simulink model "METI_Thermal_ver01_Jmaab_2018b"  (R2018b)
settings: Solver=ode8  StartTime=0  StopTime=end_time  FixedStep=sampling_time  RelTol=1e-3
PreLoadFcn:
  | %init_setting;
values from neighbouring files (symbols this model uses):
  degC2K = 273.15    [METI_TRAMI_Thermal_ver01_Jmaab_PreLoad.m]    (also in init_setting_METI.m)
  K2degC = -273.15    [METI_TRAMI_Thermal_ver01_Jmaab_PreLoad.m]    (also in init_setting_METI.m)
  sampling_time = 0.0025    [METI_TRAMI_Thermal_ver01_Jmaab_PreLoad.m]
undefined symbols (not defined in the file or in its folder): ACC_D_Gain, ACC_I_Gain, ACC_P_Gain, ALT_CNT_ALT_OFF_RPM_HYS_rpm, ALT_CNT_ALT_ON_RPM_HYS_rpm, ALT_CNT_Alter_V_BASE_V, ALT_CNT_Alter_V_Kaisei_V, ALT_CNT_flag_disable_kaisei, ALT_CNT_V_Battely_Kudo_V, ALT_PNT_ALT_GDCurrent_A, ALT_PNT_ALT_GDVolt_V, ALT_PNT_Alter_limit_Current_V_table, ALT_PNT_Alter_limit_Current_V_table_x_rpm, ALT_PNT_Alter_trq_Nm_map, ALT_PNT_Alter_trq_Nm_map_x_rpm, ALT_PNT_Alter_trq_Nm_map_y_Current_A, ALT_PNT_Alter_trq_Nm_map_z_Volt_tgt_V, ALT_PNT_eta_pulley_alt, ALT_PNT_Gain_Alt_v_del, ALT_PNT_ratio_pulley_alt, ALT_PNT_Tau_Alternator_V_tgt_s, ALT_PNT_trq_alter_output_LL_Nm, BK_PNT_Pow_UL, BK_PNT_Tau_brake, Brk_LL, Brk_PGain, Brk_UL, BT_PNT_Lo_Capa_lo_batt_F, BT_PNT_Lo_ocv_SOC_lo_batt_OCV_V_table, BT_PNT_Lo_ocv_SOC_lo_batt_OCV_V_table_x_SOC, BT_PNT_Lo_R_lo_batt_ohm, BT_PNT_Lo_SOC_MAX_lo_batt, BT_PNT_Lo_SOC_MIN_lo_batt, BT_PNT_Lo_SOC_START_lo_batt, BT_PNT_Lo_V_start_ocv, DF_PNT_DF_gear, DF_PNT_DFBlock2DFAir_Heat_Resi_KpW, DF_PNT_DFBlock_Heat_Capa_JpK, DF_PNT_DFBlock_Temp_ini_degC, DF_PNT_DFOil2DFBlock_Heat_Resi_KpW, DF_PNT_DFOil_Heat_Capa_JpK, DF_PNT_DFOil_Temp_ini_degC, DF_PNT_Driveshaft_damper, DF_PNT_Driveshaft_delta_radps_LL, DF_PNT_Driveshaft_delta_radps_UL, DF_PNT_Driveshaft_spring, DF_PNT_eta_DF, DF_PNT_Outtemp_degC, DF_PNT_TMBlock2DFBlock_Heat_Resi_KpW, Driver_Brake_Const1, Driver_Brake_Const3, Driver_Brake_Switch_Const2, Driver_Brk_sh, drivmode_ACC, drivmode_CONST, drivmode_GensokuKaisei, drivmode_GensokuRikko, drivmode_STOP, EL_PNT_R_bodyelec_lo_ohm, ENG_CNT_acc_idlestop ... (+137)
libraries: METI_Lib_vehicle_model x31, simulink x7, AZAPA_Lib_vehicle_model x1
(part 3 of 4)

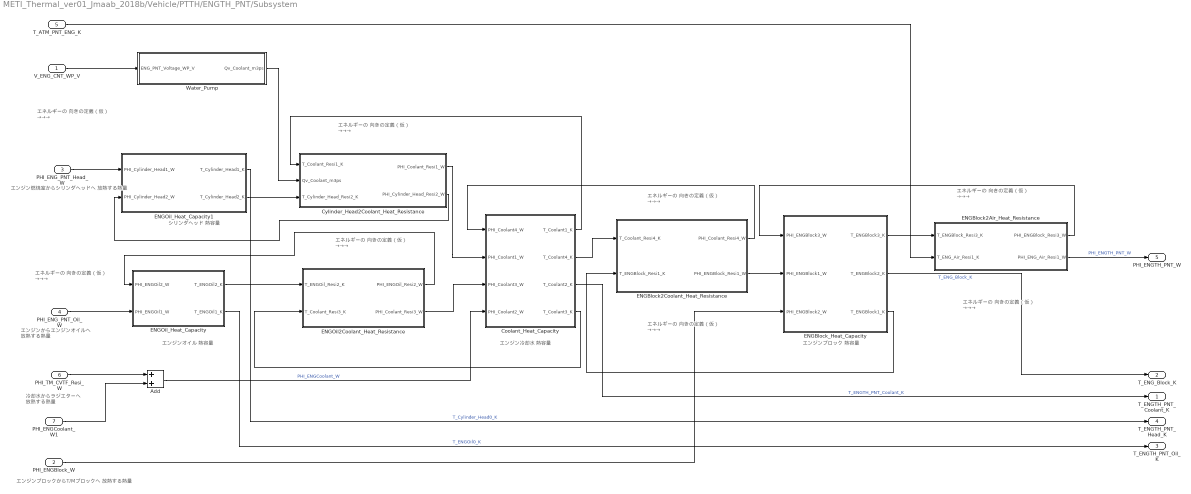
== system METI_Thermal_ver01_Jmaab_2018b/Vehicle/PTTH/ENGTH_PNT/Subsystem ==
  note: エンジンオイル
      | 熱容量
  note: エンジン冷却水
      | 熱容量
  note: エンジンブロック
      | 熱容量
  note: 冷却水からラジエターへ
      | 放熱する熱量
  note: エネルギーの
      | 向きの定義（仮）
      | →→→
  note: エンジン燃焼室からシリンダヘッドへ
      | 放熱する熱量
  note: エンジンからエンジンオイルへ
      | 放熱する熱量
  note: エネルギーの
      | 向きの定義（仮）
      | →→→
  note: エネルギーの
      | 向きの定義（仮）
      | →→→
  note: エネルギーの
      | 向きの定義（仮）
      | →→→
  note: エネルギーの
      | 向きの定義（仮）
      | →→→
  note: エネルギーの
      | 向きの定義（仮）
      | →→→
  note: エネルギーの
      | 向きの定義（仮）
      | →→→
  note: エンジンブロックからT/Mブロックへ
      | 放熱する熱量
  note: シリンダヘッド
      | 熱容量
  note: エネルギーの
      | 向きの定義（仮）
      | →→→
  V_ENG_CNT_WP_V : Inport
  PHI_ENGBlock_W : Inport  Port=2
  PHI_ENG_PNT_Head_W : Inport  Port=3
  PHI_ENG_PNT_Oil_W : Inport  Port=4
  T_ATM_PNT_ENG_K : Inport  Port=5
  PHI_TM_CVTF_Resi_W : Inport  Port=6
  PHI_ENGCoolant_W1 : Inport  Port=7
  Add : Sum
  Coolant_Heat_Capacity : Subsystem
  Cylinder_Head2Coolant_Heat_Resistance : Subsystem
  ENGBlock2Air_Heat_Resistance : Subsystem
  ENGBlock2Coolant_Heat_Resistance : Subsystem
  ENGBlock_Heat_Capacity : Subsystem
  ENGOil2Coolant_Heat_Resistance : Subsystem
  ENGOil_Heat_Capacity : Subsystem
  ENGOil_Heat_Capacity1 : Subsystem
  Water_Pump : Subsystem
  T_ENGTH_PNT_Coolant_K : Outport
  T_ENG_Block_K : Outport  Port=2
  T_ENGTH_PNT_Oil_K : Outport  Port=3
  T_ENGTH_PNT_Head_K : Outport  Port=4
  PHI_ENGTH_PNT_W : Outport  Port=5
  wires:
  PHI_TM_CVTF_Resi_W/1 -> Add/1
  Add/1 -> Coolant_Heat_Capacity/4(PHI_Coolant2_W)  "PHI_ENGCoolant_W"
  ENGOil_Heat_Capacity/1(T_ENGOil2_K) -> ENGOil2Coolant_Heat_Resistance/1(T_ENGOil_Resi2_K)
  ENGOil2Coolant_Heat_Resistance/2(PHI_Coolant_Resi3_W) -> Coolant_Heat_Capacity/3(PHI_Coolant3_W)
  PHI_ENGCoolant_W1/1 -> Add/2
  PHI_ENG_PNT_Head_W/1 -> ENGOil_Heat_Capacity1/1(PHI_Cylinder_Head1_W)
  ENGBlock_Heat_Capacity/3(T_ENGBlock1_K) -> ENGBlock2Coolant_Heat_Resistance/2(T_ENGBlock_Resi1_K)
  ENGBlock_Heat_Capacity/1(T_ENGBlock3_K) -> ENGBlock2Air_Heat_Resistance/1(T_ENGBlock_Resi3_K)
  ENGOil_Heat_Capacity1/1(T_Cylinder_Head1_K) -> T_ENGTH_PNT_Head_K/1  "T_Cylinder_Head0_K"
  Cylinder_Head2Coolant_Heat_Resistance/1(PHI_Coolant_Resi1_W) -> Coolant_Heat_Capacity/2(PHI_Coolant1_W)
  Cylinder_Head2Coolant_Heat_Resistance/2(PHI_Cylinder_Head_Resi2_W) -> ENGOil_Heat_Capacity1/2(PHI_Cylinder_Head2_W)
  Water_Pump/1(Qv_Coolant_m3ps) -> Cylinder_Head2Coolant_Heat_Resistance/2(Qv_Coolant_m3ps)
  ENGBlock_Heat_Capacity/2(T_ENGBlock2_K) -> T_ENG_Block_K/1  "T_ENG_Block_K"
  PHI_ENGBlock_W/1 -> ENGBlock_Heat_Capacity/3(PHI_ENGBlock2_W)
  V_ENG_CNT_WP_V/1 -> Water_Pump/1(ENG_PNT_Voltage_WP_V)
  ENGOil_Heat_Capacity1/2(T_Cylinder_Head2_K) -> Cylinder_Head2Coolant_Heat_Resistance/3(T_Cylinder_Head_Resi2_K)
  ENGBlock2Coolant_Heat_Resistance/1(PHI_Coolant_Resi4_W) -> Coolant_Heat_Capacity/1(PHI_Coolant4_W)
  Coolant_Heat_Capacity/4(T_Coolant3_K) -> ENGOil2Coolant_Heat_Resistance/2(T_Coolant_Resi3_K)
  ENGBlock2Air_Heat_Resistance/1(PHI_ENGBlock_Resi3_W) -> ENGBlock_Heat_Capacity/1(PHI_ENGBlock3_W)
  ENGOil2Coolant_Heat_Resistance/1(PHI_ENGOil_Resi2_W) -> ENGOil_Heat_Capacity/1(PHI_ENGOil2_W)
  Coolant_Heat_Capacity/2(T_Coolant4_K) -> ENGBlock2Coolant_Heat_Resistance/1(T_Coolant_Resi4_K)
  T_ATM_PNT_ENG_K/1 -> ENGBlock2Air_Heat_Resistance/2(T_ENG_Air_Resi1_K)
  ENGBlock2Coolant_Heat_Resistance/2(PHI_ENGBlock_Resi1_W) -> ENGBlock_Heat_Capacity/2(PHI_ENGBlock1_W)
  Coolant_Heat_Capacity/3(T_Coolant2_K) -> T_ENGTH_PNT_Coolant_K/1  "T_ENGTH_PNT_Coolant_K"
  Coolant_Heat_Capacity/1(T_Coolant1_K) -> Cylinder_Head2Coolant_Heat_Resistance/1(T_Coolant_Resi1_K)
  ENGBlock2Air_Heat_Resistance/2(PHI_ENG_Air_Resi1_W) -> PHI_ENGTH_PNT_W/1  "PHI_ENGTH_PNT_W"
  ENGOil_Heat_Capacity/2(T_ENGOil1_K) -> T_ENGTH_PNT_Oil_K/1  "T_ENGOil0_K"
  PHI_ENG_PNT_Oil_W/1 -> ENGOil_Heat_Capacity/2(PHI_ENGOil1_W)

== system METI_Thermal_ver01_Jmaab_2018b/Vehicle/PTTH/RDTH_PNT/Subsystem ==
  note: サーモスタット
  note: エネルギーの
      | 向きの定義（仮）
      | →→→
  note: エネルギーの
      | 向きの定義（仮）
      | →→→
  RD_PNT_Voltage_RDFan_V : Inport
  v_VL_PNT_kmph : Inport  Port=2
  T_ENGTH_PNT_Coolant_K : Inport  Port=3
  T_ATM_PNT_RD_K : Inport  Port=4
  ENGBlock2Coolant_Heat_Resistance : Subsystem
  RDCoolant2Air_Heat_Resistance : Subsystem
  RDCoolant_Heat_Capacity : Subsystem
  RD_Core_Heat_Resi_Calc : Subsystem
  T_RDCoolant_degC : Outport
  PHI_RDTH_PNT_W : Outport  Port=2
  PHI_RD_Air_Resi_W : Outport  Port=3
  tag scope: RD_PNT_RDCore_Heat_Resi_KpW=global
  wires:
  T_ATM_PNT_RD_K/1 -> RDCoolant2Air_Heat_Resistance/1(T_RD_Air_Resi_K)
  RDCoolant_Heat_Capacity/2(T_RDCoolant2_K) -> T_RDCoolant_degC/1, RDCoolant2Air_Heat_Resistance/3(T_RDCoolant_Resi2_K)  "T_RDCoolant_degC"
  RDCoolant_Heat_Capacity/1(T_RDCoolant1_K) -> ENGBlock2Coolant_Heat_Resistance/1(T_RDCoolant_Resi1_K)
  RD_Core_Heat_Resi_Calc/1("RD_PNT_RDCore_Heat_Resi_KpW ") -> [RD_PNT_RDCore_Heat_Resi_KpW], RDCoolant2Air_Heat_Resistance/2("RD_PNT_RDCore_Heat_Resi_KpW ")
  RDCoolant2Air_Heat_Resistance/1(PHI_RD_Air_Resi1_W) -> PHI_RD_Air_Resi_W/1  "PHI_RD_Air_Resi_W"
  T_ENGTH_PNT_Coolant_K/1 -> ENGBlock2Coolant_Heat_Resistance/2(T_Thermostat_Resi1_K)
  ENGBlock2Coolant_Heat_Resistance/2(PHI_Thermostat_Resi1_W) -> PHI_RDTH_PNT_W/1  "PHI_RDTH_PNT_W"
  RDCoolant2Air_Heat_Resistance/2(PHI_RDCoolant_Resi2_W) -> RDCoolant_Heat_Capacity/2(PHI_RDCoolant2_W)
  ENGBlock2Coolant_Heat_Resistance/1(PHI_RDCoolant_Resi1_W) -> RDCoolant_Heat_Capacity/1(PHI_RDCoolant1_W)
  RD_PNT_Voltage_RDFan_V/1 -> RD_Core_Heat_Resi_Calc/1(RD_PNT_Voltage_RDFan_V)
  v_VL_PNT_kmph/1 -> RD_Core_Heat_Resi_Calc/2(v_VL_PNT_kmph)

== system METI_Thermal_ver01_Jmaab_2018b/Vehicle/TM_PNT/DF_PNT/DriveShaft ==
  note: ドライブシャフトモデル
      | 硬いバネダンパー
  w_TR_PNT_radps : Inport
  w_DS_PNT_in_radps : Inport  Port=2
  Gain : Gain  Gain=-1
  Gain1 : Gain  Gain=DF_PNT_Driveshaft_spring
  Gain2 : Gain  Gain=DF_PNT_Driveshaft_damper
  Integrator : Integrator  LimitOutput=on  UpperSaturationLimit=DF_PNT_Driveshaft_delta_radps_UL  LowerSaturationLimit=DF_PNT_Driveshaft_delta_radps_LL
  Sum : Sum  Inputs=|+-
  Sum2 : Sum  Inputs=|++
  trq_DS_PNT_in_Nm : Outport
  trq_DF_PNT_Nm : Outport  Port=2
  wires:
  w_TR_PNT_radps/1 -> Sum/2
  w_DS_PNT_in_radps/1 -> Sum/1
  Integrator/1 -> Gain1/1
  Sum/1 -> Integrator/1, Gain2/1
  Gain1/1 -> Sum2/1
  Gain2/1 -> Sum2/2
  Sum2/1 -> Gain/1, trq_DS_PNT_in_Nm/1
  Gain/1 -> trq_DF_PNT_Nm/1

== system METI_Thermal_ver01_Jmaab_2018b/Vehicle/TM_PNT/TM_PNT/Flywheel ==
  trq_TM_PNT_in_Nm : Inport
  trq_TM_PNT_in_Nm1 : Inport  Port=2
  Divide : Product  Inputs=*/
  Inertia : Constant  Value=TM_PNT_Flywheel_Inertia_kgm2
  Integrator : Integrator  InitialCondition=TM_PNT_Flywheel_Init_radps  LimitOutput=on  LowerSaturationLimit=0
  P_cal : METI_Lib_vehicle_model/P_cal  Commented=on  Type_energy=回転運動  Type_output_energy=出力  Power_name=Po_  t_Workspace_Name=TM_PNT_Flywheel  P_VariableName=Po_TM_PNT_Flywheel  Across_VariableName=w_TM_PNT_Flywheel  Throgh_VariableName=tq_TM_PNT_Flywheel
  Sum : Sum  Inputs=|++
  Terminator : Terminator  Commented=on
  w_ENG_PNT_radps : Outport
  w_TM_PNT_in_radps : Outport  Port=2
  wires:
  Integrator/1 -> P_cal/1, w_TM_PNT_in_radps/1, w_ENG_PNT_radps/1
  trq_TM_PNT_in_Nm/1 -> Sum/1
  trq_TM_PNT_in_Nm1/1 -> Sum/2
  Inertia/1 -> Divide/2
  Sum/1 -> Divide/1, P_cal/2
  P_cal/1 -> Terminator/1
  Divide/1 -> Integrator/1

== system METI_Thermal_ver01_Jmaab_2018b/Vehicle/TM_PNT/TM_PNT/Inertia ==
  trq_TM_PNT_out_Nm0 : Inport
  trq_TM_PNT_Nm : Inport  Port=2
  Divide : Product  Inputs=*/
  Inertia : Constant  Value=TM_PNT_Driveshaft_Inertia_kgm2
  Integrator : Integrator  InitialCondition=000*(2*pi)/60  LimitOutput=on  LowerSaturationLimit=0
  P_cal : METI_Lib_vehicle_model/P_cal  Type_energy=回転運動  Type_output_energy=出力  Power_name=Po_  t_Workspace_Name=TM_PNT_inertia_MECK  P_VariableName=Po_TM_PNT_inertia_MECK  Across_VariableName=w_TM_PNT_inertia_MECK  Throgh_VariableName=tq_TM_PNT_inertia_MECK
  Sum : Sum  Inputs=|++
  Terminator : Terminator
  w_TM_PNT_out_radps : Outport
  w_TM_PNT_out_radps0 : Outport  Port=2
  wires:
  Integrator/1 -> P_cal/1, w_TM_PNT_out_radps0/1, w_TM_PNT_out_radps/1
  Divide/1 -> Integrator/1
  trq_TM_PNT_out_Nm0/1 -> Sum/1
  trq_TM_PNT_Nm/1 -> Sum/2
  Inertia/1 -> Divide/2
  Sum/1 -> Divide/1, P_cal/2
  P_cal/1 -> Terminator/1

== system METI_Thermal_ver01_Jmaab_2018b/Vehicle/TM_PNT/TM_PNT/K->degC6 ==
  K : Inport
  Constant2 : Constant  Value=K2degC
  Sum : Sum  Inputs=++|
  degC : Outport
  wires:
  K/1 -> Sum/2
  Constant2/1 -> Sum/1
  Sum/1 -> degC/1

== system METI_Thermal_ver01_Jmaab_2018b/Vehicle/TM_PNT/TM_PNT/TC_PNT ==
  note: ロックアップクラッチ
  note: トルクコンバータ
  flag_Lockup : Inport
  omg_Slip_rpm : Inport  Port=2
  w_TM_PNT_in_radps : Inport  Port=3
  w_TM_PNT_in_radps2 : Inport  Port=4
  Gain : Gain  Gain=-1
  LU_Clutch : Subsystem
  P_cal : METI_Lib_vehicle_model/P_cal  Type_energy=回転運動  Type_output_energy=出力  Power_name=Po_  t_Workspace_Name=TM_PNT_TC_MECK_UP  P_VariableName=Po_TM_PNT_TC_MECK_UP  Across_VariableName=w_TM_PNT_TC_MECK_UP  Throgh_VariableName=tq_TM_PNT_TC_MECK_UP
  P_cal1 : METI_Lib_vehicle_model/P_cal  Type_energy=回転運動  Type_output_energy=出力  Power_name=Po_  t_Workspace_Name=TM_PNT_TC_MECK_DN  P_VariableName=Po_TM_PNT_TC_MECK_DN  Across_VariableName=w_TM_PNT_TC_MECK_DN  Throgh_VariableName=tq_TM_PNT_TC_MECK_DN
  P_cal2 : METI_Lib_vehicle_model/P_cal  Type_energy=回転運動  Type_output_energy=出力  Power_name=Po_  t_Workspace_Name=TM_PNT_LU_MECK_UP  P_VariableName=Po_TM_PNT_LU_MECK_UP  Across_VariableName=w_TM_PNT_LU_MECK_UP  Throgh_VariableName=tq_TM_PNT_LU_MECK_UP
  P_cal3 : METI_Lib_vehicle_model/P_cal  Type_energy=回転運動  Type_output_energy=出力  Power_name=Po_  t_Workspace_Name=TM_PNT_LU_MECK_DN  P_VariableName=Po_TM_PNT_LU_MECK_DN  Across_VariableName=w_TM_PNT_LU_MECK_DN  Throgh_VariableName=tq_TM_PNT_LU_MECK_DN
  Sum : Sum  Inputs=|++
  Sum1 : Sum  Inputs=|++
  T_C : Subsystem
  Terminator{,1..4} (5 alike) : Terminator
  trq_TM_PNT_in_Nm2 : Outport
  trq_TM_PNT_in_Nm1 : Outport  Port=2
  wires:
  T_C/2(trq_TC_Nm2) -> Sum/2, P_cal/2
  w_TM_PNT_in_radps/1 -> T_C/1(w_TM_PNT_in_radps1), P_cal/1, LU_Clutch/2(w_TM_PNT_in_radps1), P_cal2/1
  Sum/1 -> Gain/1
  T_C/1(trq_TC_Nm1) -> P_cal1/2, Sum1/2
  Sum1/1 -> trq_TM_PNT_in_Nm2/1
  w_TM_PNT_in_radps2/1 -> LU_Clutch/3(w_TM_PNT_in_radps2), P_cal1/1, P_cal3/1, T_C/2(w_TM_PNT_in_radps2)
  P_cal/1 -> Terminator/1
  P_cal1/1 -> Terminator1/1
  omg_Slip_rpm/1 -> Terminator3/1
  LU_Clutch/1(trq_LUC_Nm1) -> Sum/1, P_cal2/2
  LU_Clutch/2(trq_LUC_Nm2) -> Sum1/1, P_cal3/2
  flag_Lockup/1 -> LU_Clutch/1(LockUP_Signal)
  P_cal2/1 -> Terminator2/1
  P_cal3/1 -> Terminator4/1
  Gain/1 -> trq_TM_PNT_in_Nm1/1

== system METI_Thermal_ver01_Jmaab_2018b/Vehicle/TM_PNT/TM_PNT/VR_PNT ==
  note: ギア比変換
  ratio_CVT : Inport
  trq_TM_PNT_in_Nm2 : Inport  Port=2
  w_TM_PNT_out_radps0 : Inport  Port=3
  T_TMTH_PNT_CVTF_dC : Inport  Port=4
  1-D Lookup Table : Lookup_n-D  NumberOfTableDimensions=1  BreakpointsForDimension1=TM_PNT_eta_CVT_x_CVTF_degC  Table=TM_PNT_eta_CVT  InternalRulePriority=Speed  RndMeth=Simplest  InputSameDT=on
  Goto1 : Goto  Commented=on  GotoTag=trq_Variator_Nm
  P_cal : METI_Lib_vehicle_model/P_cal  Type_energy=回転運動  Type_output_energy=損失  Power_name=Pl_  t_Workspace_Name=TM_PNT_Variator_MECK_LOSS  P_VariableName=Pl_TM_PNT_Variator_MECK_LOSS  Across_VariableName=w_TM_PNT_Variator_MECK_LOSS  Throgh_VariableName=tq_TM_PNT_Variator_MECK_LOSS
  Product : Product  RndMeth=Zero
  Product1 : Product  RndMeth=Zero
  Transfer Fcn : TransferFcn  Denominator=[TM_PNT_Tau_CVT_ratio_s 1]
  eta_cal_CVT : METI_Lib_vehicle_model/eta_cal_InHi  SystemSampleTime=-1
  trq_TM_PNT_out_Nm0 : Outport
  w_TM_PNT_in_radps2 : Outport  Port=2
  tag scope: tScope_CVTLoss=global
  wires:
  trq_TM_PNT_in_Nm2/1 -> eta_cal_CVT/2
  Product/1 -> w_TM_PNT_in_radps2/1, P_cal/1
  w_TM_PNT_out_radps0/1 -> Product/2
  ratio_CVT/1 -> Transfer Fcn/1
  Product1/1 -> Goto1/1, trq_TM_PNT_out_Nm0/1
  eta_cal_CVT/2 -> Product1/2
  P_cal/1 -> [tScope_CVTLoss]
  Transfer Fcn/1 -> Product1/1, Product/1
  1-D Lookup Table/1 -> eta_cal_CVT/1
  eta_cal_CVT/1 -> P_cal/2
  T_TMTH_PNT_CVTF_dC/1 -> 1-D Lookup Table/1

== system METI_Thermal_ver01_Jmaab_2018b/Driver/Caliculate_Opeining_Accel/FF/Cal_M_ENG_jiku2/Subsystem ==
  In1 : Inport
  Constant1 : Constant  Value=0
  Switch : Switch  Criteria=u2 > Threshold  Threshold=0.1
  Out1 : Outport
  wires:
  Switch/1 -> Out1/1
  Constant1/1 -> Switch/3
  In1/1 -> Switch/2, Switch/1

== system METI_Thermal_ver01_Jmaab_2018b/Vehicle/ALT_PNT/Subsystem/I_alt_cal/Cal_I_alt_P_control ==
  note: 目標電圧よりもオルタネータ電圧が低い場合電流をPI制御で出力
      | 高い場合は、電流を0とする
  V_delt_tgt : Inport
  Gain : Gain  Gain=ALT_PNT_Gain_Alt_v_del
  Transfer Fcn : TransferFcn  Denominator=[ALT_PNT_Tau_Alternator_V_tgt_s 1]
  I_alt_base : Outport
  wires:
  Gain/1 -> I_alt_base/1
  V_delt_tgt/1 -> Transfer Fcn/1
  Transfer Fcn/1 -> Gain/1

== system METI_Thermal_ver01_Jmaab_2018b/Vehicle/ALT_PNT/Subsystem/I_alt_cal/Cal_I_alt_base ==
  note: 目標電圧よりもオルタネータ電圧が低い場合電流をPI制御で出力
      | 高い場合は、電流を0とする
  V_delt_tgt : Inport
  Constant : Constant  Value=0
  Gain : Gain  Gain=1/BT_PNT_Lo_R_lo_batt_ohm
  MinMax : MinMax  Function=max  Inputs=2
  Switch : Switch  Criteria=u2 > Threshold
  Transfer Fcn : TransferFcn  Denominator=[ALT_PNT_Tau_Alternator_V_tgt_s 1]
  I_alt_base : Outport
  wires:
  MinMax/1 -> I_alt_base/1
  Gain/1 -> Switch/1
  V_delt_tgt/1 -> Transfer Fcn/1
  Constant/1 -> MinMax/2, Switch/3
  Switch/1 -> MinMax/1
  Transfer Fcn/1 -> Switch/2, Gain/1

== system METI_Thermal_ver01_Jmaab_2018b/Vehicle/CNT/ENG_CNT/ENG_Cntrl/Caliculate_Idle_Speed ==
  note: 目標アイドル回転数
  note: ○目標回転数に対するP制御
  note: 補機負荷やNDの時の負荷によるアイドル安定化処理を入れる
      | パワーデマンドで締結
  per_throttle_base : Inport
  n_eng_rpm : Inport  Port=2
  flag_Lockup : Inport  Port=3
  flag_IdleStop : Inport  Port=4
  T_ENGTH_PNT_Coolant_dC : Inport  Port=5
  Subsystem : Subsystem
  Subsystem1 : Subsystem
  Subtract : Sum  Inputs=+-
  Tw2ENG_CNT_IdleSpeed : Lookup_n-D  NumberOfTableDimensions=1  BreakpointsForDimension1=T_ENGCoodant_T_ENGCoodant  Table=ENG_CNT_IdleSpeed  InternalRulePriority=Speed  RndMeth=Simplest  InputSameDT=on
  per_isc_[%] : Outport
  tag scope: ENG_CNT_IdleSpeed=global
  wires:
  n_eng_rpm/1 -> Subsystem1/2(n_eng_rpm), Subtract/2
  Subtract/1 -> Subsystem/1(del_omg_engine)
  per_throttle_base/1 -> Subsystem1/3(per_throttle_base)
  flag_Lockup/1 -> Subsystem1/4(flag_Lockup)
  Subsystem1/1(flag_idle_fb) -> Subsystem/2(flag_idle_fb)
  flag_IdleStop/1 -> Subsystem1/5(flag_IdleStop)
  Subsystem/1(per_isc_[%]) -> per_isc_[%]/1
  T_ENGTH_PNT_Coolant_dC/1 -> Tw2ENG_CNT_IdleSpeed/1
  Tw2ENG_CNT_IdleSpeed/1 -> [ENG_CNT_IdleSpeed], Subsystem1/1(omg_tgt_idle), Subtract/1

== system METI_Thermal_ver01_Jmaab_2018b/Vehicle/CNT/ENG_CNT/ENG_Cntrl/Injection_Control ==
  T_ENGTH_PNT_Coolant_dC : Inport
  Tw2KFuel : Lookup_n-D  NumberOfTableDimensions=1  BreakpointsForDimension1=T_ENGCoodant  Table=K_Fuel  RndMeth=Simplest  InputSameDT=on
  K_Fuel : Outport
  wires:
  Tw2KFuel/1 -> K_Fuel/1  "K_Fuel"
  T_ENGTH_PNT_Coolant_dC/1 -> Tw2KFuel/1

== system METI_Thermal_ver01_Jmaab_2018b/Vehicle/CNT/ENG_CNT/ENG_Cntrl/K->degC7 ==
  K : Inport
  Constant2 : Constant  Value=K2degC
  Sum : Sum  Inputs=++|
  degC : Outport
  wires:
  Sum/1 -> degC/1
  Constant2/1 -> Sum/1
  K/1 -> Sum/2

== system METI_Thermal_ver01_Jmaab_2018b/Vehicle/CNT/ENG_CNT/ENG_Cntrl/RD_Fan_Control ==
  T_ENGTH_PNT_Coolant_dC : Inport
  1-D Lookup Table1 : Lookup_n-D  NumberOfTableDimensions=1  BreakpointsForDimension1=ENG_CNT_V_RDFan_x_T_Coolant  BeginIndexSearchUsingPreviousIndexResult=on  Table=ENG_CNT_V_RDFan_V  InternalRulePriority=Speed  RndMeth=Simplest  InputSameDT=on
  V_RDTH_PNT_Fan_V : Outport
  wires:
  T_ENGTH_PNT_Coolant_dC/1 -> 1-D Lookup Table1/1
  1-D Lookup Table1/1 -> V_RDTH_PNT_Fan_V/1

== system METI_Thermal_ver01_Jmaab_2018b/Vehicle/CNT/ENG_CNT/ENG_Cntrl/Set_Fuel_Cut ==
  note: ○減速時のフューエルカット条件
      | 　・停車中でない
      | 　・回転数がある回転数以上
      | 　・アクセル開度がOFF
  v_vehicle : Inport
  n_eng_rpm : Inport  Port=2
  per_throttle_base : Inport  Port=3
  Constant1 : Constant  Value=ENG_CNT_V_vhicle_fuelcut_kmph
  Constant4 : Constant  Value=ENG_CNT_omg_eng_fuelcut_rpm
  Constant6 : Constant  Value=ENG_CNT_per_throttle_fuelcut
  Logical Operator : Logic  Inputs=3  AllPortsSameDT=off  OutDataTypeStr=boolean
  Relational Operator1 : RelationalOperator  Operator=<=  OutDataTypeStr=boolean  RndMeth=Nearest
  Relational Operator2 : RelationalOperator  OutDataTypeStr=boolean  RndMeth=Nearest
  Relational Operator3 : RelationalOperator  OutDataTypeStr=boolean  RndMeth=Nearest
  flag_fuelcut : Outport
  wires:
  n_eng_rpm/1 -> Relational Operator2/1
  per_throttle_base/1 -> Relational Operator1/1
  Constant6/1 -> Relational Operator1/2
  Relational Operator1/1 -> Logical Operator/3
  Relational Operator2/1 -> Logical Operator/2
  Logical Operator/1 -> flag_fuelcut/1
  Constant1/1 -> Relational Operator3/2
  v_vehicle/1 -> Relational Operator3/1
  Relational Operator3/1 -> Logical Operator/1
  Constant4/1 -> Relational Operator2/2

== system METI_Thermal_ver01_Jmaab_2018b/Vehicle/CNT/ENG_CNT/ENG_Cntrl/Set_Idle_Stop ==
  note: ○アイドリングストップ制御
      | 　停車時＋ブレーキを踏んでいるとき、アイドリングストップ
  open_accel_per : Inport
  v_vehicle : Inport  Port=2
  per_brake : Inport  Port=3
  T_ENGTH_PNT_Coolant_dC : Inport  Port=4
  Constant : Constant  Value=ENG_CNT_V_car_idlestop_kmph
  Constant1 : Constant  Value=ENG_CNT_brak_idlestop
  Constant2 : Constant  Value=ENG_CNT_flag_idle_stop_exe
  Constant3 : Constant  Value=ENG_CNT_acc_idlestop
  Logical Operator : Logic  Inputs=5  AllPortsSameDT=off  OutDataTypeStr=boolean
  Relational Operator : RelationalOperator  Operator=<  OutDataTypeStr=boolean  RndMeth=Nearest
  Relational Operator1 : RelationalOperator  OutDataTypeStr=boolean  RndMeth=Nearest
  Relational Operator2 : RelationalOperator  Operator=<  OutDataTypeStr=boolean  RndMeth=Nearest
  Relay : Relay  OnSwitchValue=ENG_CNT_IdleStop_flag_const  OffSwitchValue=ENG_CNT_IdleStop_flag_const-5
  flag_IdleStop : Outport
  wires:
  Relational Operator/1 -> Logical Operator/2
  Logical Operator/1 -> flag_IdleStop/1
  v_vehicle/1 -> Relational Operator/1
  per_brake/1 -> Relational Operator1/1
  Constant/1 -> Relational Operator/2
  Constant1/1 -> Relational Operator1/2
  Relational Operator1/1 -> Logical Operator/3
  Constant2/1 -> Logical Operator/1
  T_ENGTH_PNT_Coolant_dC/1 -> Relay/1
  Relay/1 -> Logical Operator/4
  open_accel_per/1 -> Relational Operator2/1
  Constant3/1 -> Relational Operator2/2
  Relational Operator2/1 -> Logical Operator/5

== system METI_Thermal_ver01_Jmaab_2018b/Vehicle/CNT/ENG_CNT/ENG_Cntrl/Starter ==
  note: サンプリング時間
  note: 時間リセット
  note: アイドリングフラグがON→OFFに
      | 切り替わり時スターターON開始
  note: スタータ開始時間
  note: スタータ開始時間から
      | ある時間超えたらOFF
  note: アイドリングフラグがON→OFFに切り替わり時スターターON開始.ある時間を超えたらOFF
  flag_idlestop : Inport
  n_eng_rpm : Inport  Port=2
  Constant2 : Constant  Value=ENG_CNT_Starter_timer_Const_s
  Constant4 : Constant  Value=sampling_time
  Constant5 : Constant  Value=0
  Constant6 : Constant  Value=OFF
  Constant7 : Constant  Value=ON
  IdleSpeed : Constant  Value=ENG_CNT_IdleSpeed_Const/2
  Logical Operator : Logic  Inputs=3  AllPortsSameDT=off  OutDataTypeStr=boolean
  Logical Operator1 : Logic  Operator=NOT  AllPortsSameDT=off  OutDataTypeStr=boolean
  Memory : Memory  InitialCondition=1000
  Memory1 : Memory  InheritSampleTime=on
  Relational Operator1 : RelationalOperator  Operator=<=  OutDataTypeStr=boolean  RndMeth=Nearest
  Relational Operator2 : RelationalOperator  Operator=<  OutDataTypeStr=boolean  RndMeth=Nearest
  Sum5 : Sum  Inputs=|++
  Switch3 : Switch  Criteria=u2 > Threshold  Threshold=0.5
  Switch4 : Switch  Criteria=u2 > Threshold  Threshold=0.5
  flag_ON_Starter : Outport
  wires:
  Switch4/1 -> flag_ON_Starter/1
  Memory/1 -> Sum5/2
  Constant4/1 -> Sum5/1
  Constant5/1 -> Switch3/1
  Sum5/1 -> Switch3/3
  Switch3/1 -> Relational Operator1/1, Memory/1
  Memory1/1 -> Logical Operator/2
  Logical Operator1/1 -> Logical Operator/1
  flag_idlestop/1 -> Memory1/1, Logical Operator1/1
  Logical Operator/1 -> Switch3/2
  Constant2/1 -> Relational Operator1/2
  Relational Operator1/1 -> Switch4/2
  Constant7/1 -> Switch4/1
  Constant6/1 -> Switch4/3
  n_eng_rpm/1 -> Relational Operator2/1
  IdleSpeed/1 -> Relational Operator2/2
  Relational Operator2/1 -> Logical Operator/3

== system METI_Thermal_ver01_Jmaab_2018b/Vehicle/CNT/ENG_CNT/ENG_Cntrl/Water_Pump_Control ==
  T_ENGTH_PNT_Coolant_dC : Inport
  1-D Lookup Table1 : Lookup_n-D  NumberOfTableDimensions=1  BreakpointsForDimension1=ENG_CNT_V_Water_Pump_x_T_Coolant  BeginIndexSearchUsingPreviousIndexResult=on  Table=ENG_CNT_V_Water_Pump_V  InternalRulePriority=Speed  RndMeth=Simplest  InputSameDT=on
  V_ENG_PNT_WP_V : Outport
  wires:
  T_ENGTH_PNT_Coolant_dC/1 -> 1-D Lookup Table1/1
  1-D Lookup Table1/1 -> V_ENG_PNT_WP_V/1

== system METI_Thermal_ver01_Jmaab_2018b/Vehicle/CNT/TM_CNT/TM_Ctrl/CVT_ECU ==
  per_throttle : Inport
  omg_pera : Inport  Port=2
  1-D Lookup Table : Lookup_n-D  NumberOfTableDimensions=1  BreakpointsForDimension1=TM_CNT_CVTpritgt_rpm_table_x_TVO  Table=TM_CNT_CVTpritgt_rpm_table  RndMeth=Simplest  InputSameDT=on
  Constant2 : Constant  Value=TM_CNT_CVT_radpmin_min_rpm
  Divide : Product  Inputs=*/
  Gain2 : Gain  Gain=TM_CNT_Gain_CVT_ECU
  HighestRatio : Constant  Value=TM_CNT_CVT_ratio_LL
  LowestRatio : Constant  Value=TM_CNT_CVT_ratio_UL
  MinMax : MinMax  Function=max  Inputs=2
  Saturation : Saturate  UpperLimit=TM_CNT_delta_CVT_ratio_UL  LowerLimit=TM_CNT_delta_CVT_ratio_LL
  Saturation Dynamic : simulink/Discontinuities/Saturation Dynamic  OutMin=[]  OutMax=[]  OutDataTypeStr=Inherit: Same as second input  OutDataType=fixdt(1, 16)  OutScaling=2^-10  DoSatur=off
  Sum : Sum  Inputs=|+-
  Sum1 : Sum  Inputs=|++
  Unit Delay : UnitDelay  InitialCondition=1  SampleTime=-1
  ratio_CVT : Outport
  wires:
  1-D Lookup Table/1 -> Divide/1
  Divide/1 -> Saturation Dynamic/2
  LowestRatio/1 -> Saturation Dynamic/1
  HighestRatio/1 -> Saturation Dynamic/3
  MinMax/1 -> Divide/2
  Saturation Dynamic/1 -> Sum/1
  Unit Delay/1 -> Sum1/2, Sum/2
  Sum1/1 -> ratio_CVT/1, Unit Delay/1
  Sum/1 -> Gain2/1
  Gain2/1 -> Saturation/1
  per_throttle/1 -> 1-D Lookup Table/1
  omg_pera/1 -> MinMax/2
  Saturation/1 -> Sum1/1
  Constant2/1 -> MinMax/1

== system METI_Thermal_ver01_Jmaab_2018b/Vehicle/CNT/TM_CNT/TM_Ctrl/K->degC ==
  K : Inport
  Constant2 : Constant  Value=K2degC
  Sum : Sum  Inputs=++|
  degC : Outport
  wires:
  Sum/1 -> degC/1
  Constant2/1 -> Sum/1
  K/1 -> Sum/2

== system METI_Thermal_ver01_Jmaab_2018b/Vehicle/CNT/TM_CNT/TM_Ctrl/K->degC1 ==
  K : Inport
  Constant2 : Constant  Value=K2degC
  Sum : Sum  Inputs=++|
  degC : Outport
  wires:
  K/1 -> Sum/2
  Constant2/1 -> Sum/1
  Sum/1 -> degC/1

== system METI_Thermal_ver01_Jmaab_2018b/Vehicle/CNT/TM_CNT/TM_Ctrl/LockupClutch_ECU ==
  v_vehicle : Inport
  per_throttle : Inport  Port=2
  2-D Lookup Table : Lookup_n-D  BreakpointsForDimension1=TM_CNT_LU_slip_rpm_map_y_TVO  BreakpointsForDimension2=TM_CNT_LU_slip_rpm_map_x_speed_kmph  Table=TM_CNT_LU_slip_rpm_map  RndMeth=Simplest  InputSameDT=on
  Relay : Relay  OnSwitchValue=TM_CNT_LU_Clutch_RelayON_rpm  OffSwitchValue=TM_CNT_LU_Clutch_RelayOFF_rpm  OnOutputValue=0  OffOutputValue=1
  flag_Lockup : Outport
  omg_Slip_rpm : Outport  Port=2
  wires:
  v_vehicle/1 -> 2-D Lookup Table/2
  2-D Lookup Table/1 -> omg_Slip_rpm/1, Relay/1
  per_throttle/1 -> 2-D Lookup Table/1
  Relay/1 -> flag_Lockup/1

== system METI_Thermal_ver01_Jmaab_2018b/Vehicle/CNT/TM_CNT/TM_Ctrl/WarmerECU ==
  note: ENG冷却水温＞CVTF温度
      | の時にこのマップを使用する
  note: CVTF温度が熱い時に
      | このマップを使用する
  T_TMTH_PNT_CVTF_dC : Inport
  T_ENG_Coolant_dC : Inport  Port=2
  1-D Lookup Table1 : Lookup_n-D  NumberOfTableDimensions=1  BreakpointsForDimension1=TM_CNT_CVTFwarmer_KpW_x_T_ENGCoolant  BeginIndexSearchUsingPreviousIndexResult=on  Table=TM_CNT_CVTFwarmer_KpW  ExtrapMethod=Clip  InternalRulePriority=Speed  RndMeth=Simplest  InputSameDT=on
  1-D Lookup Table2 : Lookup_n-D  NumberOfTableDimensions=1  BreakpointsForDimension1=TM_CNT_CVTFwarmer2_KpW_x_T_CVTF  BeginIndexSearchUsingPreviousIndexResult=on  Table=TM_CNT_CVTFwarmer2_KpW  ExtrapMethod=Clip  InternalRulePriority=Speed  RndMeth=Simplest  InputSameDT=on
  Add1 : Sum  Inputs=+-
  Compare To Zero1 : simulink/Logic and Bit Operations/Compare To Zero  relop=>  OutDataTypeStr=boolean
  Constant1 : Constant  Value=TM_CNT_CVTFwarmer_cold_Coolant_KpW
  MinMax : MinMax  Inputs=2
  Switch1 : Switch  Criteria=u2 > Threshold
  R_CVTF_warmer_tgt_KpW : Outport
  wires:
  MinMax/1 -> R_CVTF_warmer_tgt_KpW/1
  Add1/1 -> Compare To Zero1/1
  Compare To Zero1/1 -> Switch1/2
  1-D Lookup Table1/1 -> Switch1/1
  Constant1/1 -> Switch1/3
  T_ENG_Coolant_dC/1 -> 1-D Lookup Table1/1, Add1/1
  T_TMTH_PNT_CVTF_dC/1 -> 1-D Lookup Table2/1, Add1/2
  Switch1/1 -> MinMax/1
  1-D Lookup Table2/1 -> MinMax/2

== system METI_Thermal_ver01_Jmaab_2018b/Vehicle/ENG_PNT/ENG_Plant/Cal_FuelComsunption/Not_cal1 ==
  In1 : Inport
  Constant : Constant  Value=0
  Constant1 : Constant
  Switch : Switch  Criteria=u2 > Threshold  Threshold=0.5
  Out1 : Outport
  wires:
  Constant1/1 -> Switch/3
  Constant/1 -> Switch/1
  Switch/1 -> Out1/1
  In1/1 -> Switch/2

== system METI_Thermal_ver01_Jmaab_2018b/Vehicle/ENG_PNT/ENG_Plant/Cal_FuelComsunption/Not_cal2 ==
  In1 : Inport
  Constant : Constant  Value=0
  Constant1 : Constant
  Switch : Switch  Criteria=u2 > Threshold  Threshold=0.5
  Out1 : Outport
  wires:
  In1/1 -> Switch/2
  Switch/1 -> Out1/1
  Constant/1 -> Switch/1
  Constant1/1 -> Switch/3

== system METI_Thermal_ver01_Jmaab_2018b/Vehicle/ENG_PNT/ENG_Plant/Cal_trq_ENG_jiku/Not_cal ==
  In1 : Inport
  Constant : Constant  Value=0
  Constant1 : Constant
  Switch : Switch  Criteria=u2 > Threshold  Threshold=0.5
  Out1 : Outport
  wires:
  In1/1 -> Switch/2
  Switch/1 -> Out1/1
  Constant/1 -> Switch/1
  Constant1/1 -> Switch/3

== system METI_Thermal_ver01_Jmaab_2018b/Vehicle/ENG_PNT/ENG_Plant/Cal_trq_ENG_jiku/Not_cal1 ==
  In1 : Inport
  Constant : Constant  Value=0
  Constant1 : Constant
  Switch : Switch  Criteria=u2 > Threshold  Threshold=0.5
  Out1 : Outport
  wires:
  Constant1/1 -> Switch/3
  Constant/1 -> Switch/1
  Switch/1 -> Out1/1
  In1/1 -> Switch/2

== system METI_Thermal_ver01_Jmaab_2018b/Vehicle/PTTH/DTTH_PNT/DFTH_PNT/DFBlock_Heat_Capacity ==
  PHI_DFBlock3_W : Inport
  PHI_DFBlock2_W : Inport  Port=2
  PHI_DFBlock1_W : Inport  Port=3
  Add : Sum  Inputs=+++
  Add1 : Sum
  Constant : Constant  Value=DF_PNT_DFBlock_Heat_Capa_JpK
  Constant1 : Constant  Value=DF_PNT_DFBlock_Temp_ini_degC
  Divide : Product  Inputs=/*
  Integrator : Integrator
  degC->K : Subsystem
  T_DFBlock2_K : Outport
  T_DFBlock3_K : Outport  Port=2
  T_DFBlock1_K : Outport  Port=3
  wires:
  PHI_DFBlock1_W/1 -> Add/1
  Constant/1 -> Divide/1
  Add/1 -> Divide/2
  Divide/1 -> Integrator/1
  Integrator/1 -> Add1/2
  Add1/1 -> T_DFBlock1_K/1, T_DFBlock3_K/1, T_DFBlock2_K/1
  PHI_DFBlock2_W/1 -> Add/2
  PHI_DFBlock3_W/1 -> Add/3
  Constant1/1 -> degC->K/1(degC)
  degC->K/1(K) -> Add1/1

== system METI_Thermal_ver01_Jmaab_2018b/Vehicle/PTTH/DTTH_PNT/DFTH_PNT/DFOil2DFBlock_Heat_Resistance ==
  T_DFOil_Resi2_K : Inport
  T_DFBlock_Resi_K : Inport  Port=2
  Add : Sum  Inputs=+-
  Constant : Constant  Value=DF_PNT_DFOil2DFBlock_Heat_Resi_KpW
  Divide : Product  Inputs=*/
  Gain : Gain  Gain=-1
  Gain1 : Gain
  PHI_DFOil_Resi2_W : Outport
  PHI_DFBlock_Resi_W : Outport  Port=2
  wires:
  Constant/1 -> Divide/2
  Add/1 -> Divide/1
  Divide/1 -> Gain/1, Gain1/1
  Gain/1 -> PHI_DFOil_Resi2_W/1
  T_DFOil_Resi2_K/1 -> Add/1
  T_DFBlock_Resi_K/1 -> Add/2
  Gain1/1 -> PHI_DFBlock_Resi_W/1

== system METI_Thermal_ver01_Jmaab_2018b/Vehicle/PTTH/DTTH_PNT/DFTH_PNT/DFOil_Heat_Capacity ==
  PHI_DFOil2_W : Inport
  PHI_DFOil1_W : Inport  Port=2
  Add : Sum
  Add1 : Sum
  Constant : Constant  Value=DF_PNT_DFOil_Heat_Capa_JpK
  Constant1 : Constant  Value=DF_PNT_DFOil_Temp_ini_degC
  Divide : Product  Inputs=/*
  Integrator : Integrator
  degC->K : Subsystem
  T_DFOil2_K : Outport
  T_DFOil1_K : Outport  Port=2
  wires:
  PHI_DFOil2_W/1 -> Add/2
  PHI_DFOil1_W/1 -> Add/1
  Constant/1 -> Divide/1
  Add/1 -> Divide/2
  Divide/1 -> Integrator/1
  Integrator/1 -> Add1/2
  Add1/1 -> T_DFOil1_K/1, T_DFOil2_K/1
  Constant1/1 -> degC->K/1(degC)
  degC->K/1(K) -> Add1/1

== system METI_Thermal_ver01_Jmaab_2018b/Vehicle/PTTH/DTTH_PNT/DFTH_PNT/ENGBlock2Air_Heat_Resistance ==
  T_DFBlock_Resi_K : Inport
  T_DF_Air_Resi_K : Inport  Port=2
  Add : Sum  Inputs=+-
  Constant : Constant  Value=DF_PNT_DFBlock2DFAir_Heat_Resi_KpW
  Divide : Product  Inputs=*/
  Gain : Gain  Gain=-1
  Gain1 : Gain
  PHI_DFBlock_Resi_W : Outport
  PHI_DF_Air_Resi_W : Outport  Port=2
  wires:
  Constant/1 -> Divide/2
  Add/1 -> Divide/1
  Divide/1 -> Gain/1, Gain1/1
  Gain/1 -> PHI_DFBlock_Resi_W/1
  T_DFBlock_Resi_K/1 -> Add/1
  T_DF_Air_Resi_K/1 -> Add/2
  Gain1/1 -> PHI_DF_Air_Resi_W/1

== system METI_Thermal_ver01_Jmaab_2018b/Vehicle/PTTH/DTTH_PNT/DFTH_PNT/TMBlock2DFBlock_Heat_Resistance ==
  T_DFBlock_Resi_K : Inport
  T_TMBlock_Resi_K : Inport  Port=2
  Add : Sum  Inputs=+-
  Constant : Constant  Value=DF_PNT_TMBlock2DFBlock_Heat_Resi_KpW
  Divide : Product  Inputs=*/
  Gain : Gain  Gain=-1
  Gain1 : Gain
  PHI_DFBlock_Resi_W : Outport
  PHI_TMBlock_Resi_W : Outport  Port=2
  wires:
  Constant/1 -> Divide/2
  Add/1 -> Divide/1
  Divide/1 -> Gain/1, Gain1/1
  Gain/1 -> PHI_TMBlock_Resi_W/1
  T_TMBlock_Resi_K/1 -> Add/1
  T_DFBlock_Resi_K/1 -> Add/2
  Gain1/1 -> PHI_DFBlock_Resi_W/1

== system METI_Thermal_ver01_Jmaab_2018b/Vehicle/PTTH/DTTH_PNT/TMTH_PNT/CVTF2Coolant_Heat_Resistance ==
  note: エネルギーの
      | 向きの定義（仮）
      | ← ←←
  T_CVTF_Resi2_K : Inport
  R_CVTF_warmer_tgt_KpW : Inport  Port=2
  T_Coolant_Resi2_K : Inport  Port=3
  Add : Sum  Inputs=+-
  Divide : Product  Inputs=*/
  Gain : Gain  Gain=-1
  Gain1 : Gain  Gain=-1
  PHI_Coolant_Resi2_W : Outport
  PHI_CVTF_Resi2_W : Outport  Port=2
  wires:
  R_CVTF_warmer_tgt_KpW/1 -> Divide/2
  Add/1 -> Divide/1
  Divide/1 -> Gain/1, Gain1/1
  T_Coolant_Resi2_K/1 -> Add/2
  T_CVTF_Resi2_K/1 -> Add/1
  Gain/1 -> PHI_CVTF_Resi2_W/1
  Gain1/1 -> PHI_Coolant_Resi2_W/1

== system METI_Thermal_ver01_Jmaab_2018b/Vehicle/PTTH/DTTH_PNT/TMTH_PNT/CVTF2TMBlock_Heat_Resistance ==
  T_CVTF_Resi4_K : Inport
  T_TMBlock_Resi1_K : Inport  Port=2
  Add : Sum  Inputs=+-
  Constant : Constant  Value=TM_PNT_CVTF2TMBlock_Heat_Resi_KpW
  Divide : Product  Inputs=*/
  Gain : Gain  Gain=-1
  Gain1 : Gain
  PHI_CVTF_Resi4_W : Outport
  PHI_TMBlock_Resi1_W : Outport  Port=2
  wires:
  Constant/1 -> Divide/2
  Add/1 -> Divide/1
  Divide/1 -> Gain/1, Gain1/1
  Gain/1 -> PHI_CVTF_Resi4_W/1
  T_CVTF_Resi4_K/1 -> Add/1
  T_TMBlock_Resi1_K/1 -> Add/2
  Gain1/1 -> PHI_TMBlock_Resi1_W/1

== system METI_Thermal_ver01_Jmaab_2018b/Vehicle/PTTH/DTTH_PNT/TMTH_PNT/CVTF_Heat_Capacity ==
  PHI_CVTF4_W : Inport
  PHI_CVTF1_W : Inport  Port=2
  PHI_CVT2_W : Inport  Port=3
  Add : Sum  Inputs=+++
  Add1 : Sum
  Constant : Constant  Value=TM_PNT_CVTF_Heat_Capa_JpK
  Constant1 : Constant  Value=TM_PNT_CVTF_Temp_ini_degC
  Divide : Product  Inputs=/*
  Integrator : Integrator
  degC->K : Subsystem
  T_CVTF4_K : Outport
  T_CVTF2_K : Outport  Port=2
  T_CVTF1_K : Outport  Port=3
  wires:
  PHI_CVT2_W/1 -> Add/3
  PHI_CVTF1_W/1 -> Add/1
  Constant/1 -> Divide/1
  Add/1 -> Divide/2
  Divide/1 -> Integrator/1
  Integrator/1 -> Add1/2
  Add1/1 -> T_CVTF1_K/1, T_CVTF2_K/1, T_CVTF4_K/1
  PHI_CVTF4_W/1 -> Add/2
  Constant1/1 -> degC->K/1(degC)
  degC->K/1(K) -> Add1/1

== system METI_Thermal_ver01_Jmaab_2018b/Vehicle/PTTH/DTTH_PNT/TMTH_PNT/ENGBlock2TMBlock_Heat_Resistance ==
  T_TMBlock_Resi2_K : Inport
  T_ENGBlock_Resi2_K : Inport  Port=2
  Add : Sum  Inputs=+-
  Constant : Constant  Value=TM_PNT_ENGBlock2TMBlock_Heat_Resi_KpW
  Divide : Product  Inputs=*/
  Gain : Gain  Gain=-1
  Gain1 : Gain
  PHI_TMBlock_Resi2_W : Outport
  PHI_ENGBlock_Resi2_W : Outport  Port=2
  wires:
  Constant/1 -> Divide/2
  Add/1 -> Divide/1
  Divide/1 -> Gain1/1, Gain/1
  Gain/1 -> PHI_ENGBlock_Resi2_W/1
  T_ENGBlock_Resi2_K/1 -> Add/1
  T_TMBlock_Resi2_K/1 -> Add/2
  Gain1/1 -> PHI_TMBlock_Resi2_W/1

== system METI_Thermal_ver01_Jmaab_2018b/Vehicle/PTTH/DTTH_PNT/TMTH_PNT/TMBlock2Air_Heat_Resistance ==
  T_TMBlock_Resi3_K : Inport
  T_TM_Air_Resi1_K : Inport  Port=2
  Add : Sum  Inputs=+-
  Constant : Constant  Value=TM_PNT_TMBlock2TMAir_Heat_Resi_KpW
  Divide : Product  Inputs=*/
  Gain : Gain  Gain=-1
  Gain1 : Gain
  PHI_TMBlock_Resi3_W : Outport
  PHI_TM_Air_Resi1_W : Outport  Port=2
  wires:
  Constant/1 -> Divide/2
  Add/1 -> Divide/1
  Divide/1 -> Gain/1, Gain1/1
  Gain/1 -> PHI_TMBlock_Resi3_W/1
  T_TMBlock_Resi3_K/1 -> Add/1
  T_TM_Air_Resi1_K/1 -> Add/2
  Gain1/1 -> PHI_TM_Air_Resi1_W/1

== system METI_Thermal_ver01_Jmaab_2018b/Vehicle/PTTH/DTTH_PNT/TMTH_PNT/TMBlock_Heat_Capacity ==
  PHI_TMBlock3_W : Inport
  PHI_TMBlock2_W : Inport  Port=2
  PHI_TMBlock1_W : Inport  Port=3
  PHI_TMBlock4_W : Inport  Port=4
  Add : Sum  Inputs=++++
  Add1 : Sum
  Constant : Constant  Value=TM_PNT_TMBlock_Heat_Capa_JpK
  Constant1 : Constant  Value=TM_PNT_TMBlock_Temp_ini_degC
  Divide : Product  Inputs=/*
  Integrator : Integrator
  degC->K : Subsystem
  T_TMBlock2_K : Outport
  T_TMBlock3_K : Outport  Port=2
  T_TMBlock4_K : Outport  Port=3
  T_TMBlock1_K : Outport  Port=4
  wires:
  PHI_TMBlock2_W/1 -> Add/4
  PHI_TMBlock1_W/1 -> Add/1
  Constant/1 -> Divide/1
  Add/1 -> Divide/2
  Divide/1 -> Integrator/1
  Integrator/1 -> Add1/2
  PHI_TMBlock3_W/1 -> Add/3
  PHI_TMBlock4_W/1 -> Add/2
  Add1/1 -> T_TMBlock1_K/1, T_TMBlock4_K/1, T_TMBlock3_K/1, T_TMBlock2_K/1
  Constant1/1 -> degC->K/1(degC)
  degC->K/1(K) -> Add1/1

== system METI_Thermal_ver01_Jmaab_2018b/Vehicle/PTTH/ENGTH_PNT/Subsystem/Coolant_Heat_Capacity ==
  PHI_Coolant4_W : Inport
  PHI_Coolant1_W : Inport  Port=2
  PHI_Coolant3_W : Inport  Port=3
  PHI_Coolant2_W : Inport  Port=4
  Add : Sum  Inputs=++++
  Add1 : Sum
  Constant : Constant  Value=ENG_PNT_Coolant_Heat_Capa_JpK
  Constant1 : Constant  Value=ENG_PNT_Coolant_Temp_ini_degC
  Divide : Product  Inputs=/*
  Integrator : Integrator
  degC->K : Subsystem
  T_Coolant1_K : Outport
  T_Coolant4_K : Outport  Port=2
  T_Coolant2_K : Outport  Port=3
  T_Coolant3_K : Outport  Port=4
  wires:
  PHI_Coolant2_W/1 -> Add/4
  PHI_Coolant1_W/1 -> Add/1
  Constant/1 -> Divide/1
  Add/1 -> Divide/2
  Divide/1 -> Integrator/1
  Integrator/1 -> Add1/2
  Add1/1 -> T_Coolant3_K/1, T_Coolant2_K/1, T_Coolant4_K/1, T_Coolant1_K/1
  PHI_Coolant3_W/1 -> Add/2
  PHI_Coolant4_W/1 -> Add/3
  degC->K/1(K) -> Add1/1
  Constant1/1 -> degC->K/1(degC)

== system METI_Thermal_ver01_Jmaab_2018b/Vehicle/PTTH/ENGTH_PNT/Subsystem/Cylinder_Head2Coolant_Heat_Resistance ==
  T_Coolant_Resi1_K : Inport
  Qv_Coolant_m3ps : Inport  Port=2
  T_Cylinder_Head_Resi2_K : Inport  Port=3
  1-D Lookup Table : Lookup_n-D  NumberOfTableDimensions=1  BreakpointsForDimension1=ENG_PNT_Cylinder_Head2Coolant_Heat_Resi_x_qv_Coolant  Table=ENG_PNT_Cylinder_Head2Coolant_Heat_Resi_KpW  InternalRulePriority=Speed  RndMeth=Simplest  InputSameDT=on
  Add : Sum  Inputs=+-
  Divide : Product  Inputs=*/
  Gain : Gain  Gain=-1
  Gain1 : Gain
  PHI_Coolant_Resi1_W : Outport
  PHI_Cylinder_Head_Resi2_W : Outport  Port=2
  wires:
  T_Cylinder_Head_Resi2_K/1 -> Add/1
  T_Coolant_Resi1_K/1 -> Add/2
  1-D Lookup Table/1 -> Divide/2
  Add/1 -> Divide/1
  Divide/1 -> Gain/1, Gain1/1
  Gain/1 -> PHI_Cylinder_Head_Resi2_W/1
  Gain1/1 -> PHI_Coolant_Resi1_W/1
  Qv_Coolant_m3ps/1 -> 1-D Lookup Table/1

== system METI_Thermal_ver01_Jmaab_2018b/Vehicle/PTTH/ENGTH_PNT/Subsystem/ENGBlock2Air_Heat_Resistance ==
  T_ENGBlock_Resi3_K : Inport
  T_ENG_Air_Resi1_K : Inport  Port=2
  Add : Sum  Inputs=+-
  Constant : Constant  Value=ENG_PNT_ENGBlock2ENGAir_Heat_Resi_KpW
  Divide : Product  Inputs=*/
  Gain : Gain  Gain=-1
  Gain1 : Gain
  PHI_ENGBlock_Resi3_W : Outport
  PHI_ENG_Air_Resi1_W : Outport  Port=2
  wires:
  Constant/1 -> Divide/2
  Add/1 -> Divide/1
  Divide/1 -> Gain1/1, Gain/1
  Gain/1 -> PHI_ENGBlock_Resi3_W/1
  T_ENGBlock_Resi3_K/1 -> Add/1
  T_ENG_Air_Resi1_K/1 -> Add/2
  Gain1/1 -> PHI_ENG_Air_Resi1_W/1

== system METI_Thermal_ver01_Jmaab_2018b/Vehicle/PTTH/ENGTH_PNT/Subsystem/ENGBlock2Coolant_Heat_Resistance ==
  T_Coolant_Resi4_K : Inport
  T_ENGBlock_Resi1_K : Inport  Port=2
  Add : Sum  Inputs=+-
  Constant : Constant  Value=ENG_PNT_Coolant2ENGBlock_Heat_Resi_KpW
  Divide : Product  Inputs=*/
  Gain : Gain  Gain=-1
  Gain1 : Gain
  PHI_Coolant_Resi4_W : Outport
  PHI_ENGBlock_Resi1_W : Outport  Port=2
  wires:
  Constant/1 -> Divide/2
  Add/1 -> Divide/1
  Divide/1 -> Gain1/1, Gain/1
  Gain/1 -> PHI_Coolant_Resi4_W/1
  T_Coolant_Resi4_K/1 -> Add/1
  T_ENGBlock_Resi1_K/1 -> Add/2
  Gain1/1 -> PHI_ENGBlock_Resi1_W/1

== system METI_Thermal_ver01_Jmaab_2018b/Vehicle/PTTH/ENGTH_PNT/Subsystem/ENGBlock_Heat_Capacity ==
  PHI_ENGBlock3_W : Inport
  PHI_ENGBlock1_W : Inport  Port=2
  PHI_ENGBlock2_W : Inport  Port=3
  Add : Sum  Inputs=+++
  Add1 : Sum
  Constant : Constant  Value=ENG_PNT_ENGBlock_Heat_Capa_JpK
  Constant1 : Constant  Value=ENG_PNT_ENGBlock_Temp_ini_degC
  Divide : Product  Inputs=/*
  Integrator : Integrator
  degC->K : Subsystem
  T_ENGBlock3_K : Outport
  T_ENGBlock2_K : Outport  Port=2
  T_ENGBlock1_K : Outport  Port=3
  wires:
  PHI_ENGBlock2_W/1 -> Add/3
  PHI_ENGBlock1_W/1 -> Add/1
  Constant/1 -> Divide/1
  Add/1 -> Divide/2
  Divide/1 -> Integrator/1
  Integrator/1 -> Add1/2
  Add1/1 -> T_ENGBlock2_K/1, T_ENGBlock1_K/1, T_ENGBlock3_K/1
  PHI_ENGBlock3_W/1 -> Add/2
  Constant1/1 -> degC->K/1(degC)
  degC->K/1(K) -> Add1/1

== system METI_Thermal_ver01_Jmaab_2018b/Vehicle/PTTH/ENGTH_PNT/Subsystem/ENGOil2Coolant_Heat_Resistance ==
  T_ENGOil_Resi2_K : Inport
  T_Coolant_Resi3_K : Inport  Port=2
  Add : Sum  Inputs=+-
  Constant : Constant  Value=ENG_PNT_ENGOil2Coolant_Heat_Resi_KpW
  Divide : Product  Inputs=*/
  Gain : Gain  Gain=-1
  Gain1 : Gain
  PHI_ENGOil_Resi2_W : Outport
  PHI_Coolant_Resi3_W : Outport  Port=2
  wires:
  T_ENGOil_Resi2_K/1 -> Add/1
  T_Coolant_Resi3_K/1 -> Add/2
  Constant/1 -> Divide/2
  Add/1 -> Divide/1
  Divide/1 -> Gain/1, Gain1/1
  Gain/1 -> PHI_ENGOil_Resi2_W/1
  Gain1/1 -> PHI_Coolant_Resi3_W/1

== system METI_Thermal_ver01_Jmaab_2018b/Vehicle/PTTH/ENGTH_PNT/Subsystem/ENGOil_Heat_Capacity ==
  PHI_ENGOil2_W : Inport
  PHI_ENGOil1_W : Inport  Port=2
  Add : Sum
  Add1 : Sum
  Constant : Constant  Value=ENG_PNT_ENGOil_Heat_Capa_JpK
  Constant1 : Constant  Value=ENG_PNT_ENGOil_Temp_ini_degC
  Divide : Product  Inputs=/*
  Integrator : Integrator
  degC->K : Subsystem
  T_ENGOil2_K : Outport
  T_ENGOil1_K : Outport  Port=2
  wires:
  PHI_ENGOil2_W/1 -> Add/2
  PHI_ENGOil1_W/1 -> Add/1
  Constant/1 -> Divide/1
  Add/1 -> Divide/2
  Divide/1 -> Integrator/1
  Integrator/1 -> Add1/2
  Add1/1 -> T_ENGOil2_K/1, T_ENGOil1_K/1
  Constant1/1 -> degC->K/1(degC)
  degC->K/1(K) -> Add1/1

== system METI_Thermal_ver01_Jmaab_2018b/Vehicle/PTTH/ENGTH_PNT/Subsystem/ENGOil_Heat_Capacity1 ==
  PHI_Cylinder_Head1_W : Inport
  PHI_Cylinder_Head2_W : Inport  Port=2
  Add : Sum
  Add1 : Sum
  Constant : Constant  Value=ENG_PNT_Cylinder_Head_Heat_Capa_JpK
  Constant1 : Constant  Value=ENG_PNT_Cylinder_Head_Temp_ini_degC
  Divide : Product  Inputs=/*
  Integrator : Integrator
  degC->K : Subsystem
  T_Cylinder_Head1_K : Outport
  T_Cylinder_Head2_K : Outport  Port=2
  wires:
  PHI_Cylinder_Head2_W/1 -> Add/2
  PHI_Cylinder_Head1_W/1 -> Add/1
  Constant/1 -> Divide/1
  Add/1 -> Divide/2
  Divide/1 -> Integrator/1
  Integrator/1 -> Add1/2
  Add1/1 -> T_Cylinder_Head2_K/1, T_Cylinder_Head1_K/1
  Constant1/1 -> degC->K/1(degC)
  degC->K/1(K) -> Add1/1

== system METI_Thermal_ver01_Jmaab_2018b/Vehicle/PTTH/ENGTH_PNT/Subsystem/Water_Pump ==
  ENG_PNT_Voltage_WP_V : Inport
  1-D Lookup Table : Lookup_n-D  NumberOfTableDimensions=1  BreakpointsForDimension1=ENG_PNT_Qv_Water_Pump_x_V_WP  Table=ENG_PNT_Qv_Water_Pump_m3ps  InternalRulePriority=Speed  RndMeth=Simplest  InputSameDT=on
  Qv_Coolant_m3ps : Outport
  wires:
  ENG_PNT_Voltage_WP_V/1 -> 1-D Lookup Table/1
  1-D Lookup Table/1 -> Qv_Coolant_m3ps/1

== system METI_Thermal_ver01_Jmaab_2018b/Vehicle/PTTH/RDTH_PNT/Subsystem/ENGBlock2Coolant_Heat_Resistance ==
  T_RDCoolant_Resi1_K : Inport
  T_Thermostat_Resi1_K : Inport  Port=2
  1-D Lookup Table : Lookup_n-D  NumberOfTableDimensions=1  BreakpointsForDimension1=RD_PNT_Thermostat_Heat_Resi_KpW_T_Coolant  Table=RD_PNT_Thermostat_Heat_Resi_KpW  InternalRulePriority=Speed  RndMeth=Simplest  InputSameDT=on
  Add : Sum  Inputs=+-
  Divide : Product  Inputs=*/
  Gain : Gain  Gain=-1
  Gain1 : Gain
  K->degC : Subsystem
  PHI_RDCoolant_Resi1_W : Outport
  PHI_Thermostat_Resi1_W : Outport  Port=2
  tag scope: RD_PNT_Thermostat_Heat_Resi_KpW=global
  wires:
  Add/1 -> Divide/1
  Divide/1 -> Gain/1, Gain1/1
  Gain/1 -> PHI_Thermostat_Resi1_W/1
  T_Thermostat_Resi1_K/1 -> Add/1, K->degC/1(K)
  T_RDCoolant_Resi1_K/1 -> Add/2
  Gain1/1 -> PHI_RDCoolant_Resi1_W/1
  K->degC/1(degC) -> 1-D Lookup Table/1
  1-D Lookup Table/1 -> [RD_PNT_Thermostat_Heat_Resi_KpW], Divide/2

== system METI_Thermal_ver01_Jmaab_2018b/Vehicle/PTTH/RDTH_PNT/Subsystem/RDCoolant2Air_Heat_Resistance ==
  T_RD_Air_Resi_K : Inport
  "RD_PNT_RDCore_Heat_Resi_KpW " : Inport  Port=2
  T_RDCoolant_Resi2_K : Inport  Port=3
  Add : Sum  Inputs=+-
  Divide : Product  Inputs=*/
  Gain : Gain  Gain=-1
  Gain1 : Gain
  PHI_RD_Air_Resi1_W : Outport
  PHI_RDCoolant_Resi2_W : Outport  Port=2
  wires:
  "RD_PNT_RDCore_Heat_Resi_KpW "/1 -> Divide/2
  Add/1 -> Divide/1
  Divide/1 -> Gain/1, Gain1/1
  Gain/1 -> PHI_RDCoolant_Resi2_W/1
  T_RDCoolant_Resi2_K/1 -> Add/1
  T_RD_Air_Resi_K/1 -> Add/2
  Gain1/1 -> PHI_RD_Air_Resi1_W/1

== system METI_Thermal_ver01_Jmaab_2018b/Vehicle/PTTH/RDTH_PNT/Subsystem/RDCoolant_Heat_Capacity ==
  PHI_RDCoolant1_W : Inport
  PHI_RDCoolant2_W : Inport  Port=2
  Add : Sum
  Add1 : Sum
  Constant : Constant  Value=RD_PNT_RDCoolant_Heat_Capa_JpK
  Constant1 : Constant  Value=RD_PNT_RDCoolant_Temp_ini_degC
  Divide : Product  Inputs=/*
  Integrator : Integrator
  degC->K : Subsystem
  T_RDCoolant1_K : Outport
  T_RDCoolant2_K : Outport  Port=2
  wires:
  PHI_RDCoolant2_W/1 -> Add/2
  PHI_RDCoolant1_W/1 -> Add/1
  Constant/1 -> Divide/1
  Add/1 -> Divide/2
  Divide/1 -> Integrator/1
  Integrator/1 -> Add1/2
  Add1/1 -> T_RDCoolant2_K/1, T_RDCoolant1_K/1
  Constant1/1 -> degC->K/1(degC)
  degC->K/1(K) -> Add1/1

== system METI_Thermal_ver01_Jmaab_2018b/Vehicle/PTTH/RDTH_PNT/Subsystem/RD_Core_Heat_Resi_Calc ==
  note: ラジエターファンの動作で
      | 発生する風速
  note: 車両の走行によって
      | ラジエターグリルに発生する風速
  note: ラジエターファンの動作で
      | ラジエターコアに当たる風量
  note: 車両の走行によって
      | ラジエターコアに当たる風量
  RD_PNT_Voltage_RDFan_V : Inport
  v_VL_PNT_kmph : Inport  Port=2
  1-D Lookup Table : Lookup_n-D  NumberOfTableDimensions=1  BreakpointsForDimension1=RD_PNT_RDCore_Heat_Resi_KpW_x_Wind_m3ps  Table=RD_PNT_RDCore_Heat_Resi_KpW  InternalRulePriority=Speed  RndMeth=Simplest  InputSameDT=on
  1-D Lookup Table1 : Lookup_n-D  NumberOfTableDimensions=1  BreakpointsForDimension1=RD_PNT_v_RDFan_Wind_vel_mps_x_V_RDFan  Table=RD_PNT_v_RDFan_Wind_vel_mps  InternalRulePriority=Speed  RndMeth=Simplest  InputSameDT=on
  Abs : Abs
  Add : Sum
  Constant : Constant  Value=RD_PNT_RDFan_area_m2
  Constant1 : Constant  Value=RD_PNT_RDGrill_area_m2
  Product : Product
  Product1 : Product
  gain1 : Gain  Gain=kmph2mps
  "RD_PNT_RDCore_Heat_Resi_KpW " : Outport
  wires:
  RD_PNT_Voltage_RDFan_V/1 -> 1-D Lookup Table1/1
  Constant/1 -> Product/2
  v_VL_PNT_kmph/1 -> gain1/1
  Constant1/1 -> Product1/2
  Product/1 -> Add/1
  Product1/1 -> Add/2
  Add/1 -> Abs/1
  1-D Lookup Table/1 -> "RD_PNT_RDCore_Heat_Resi_KpW "/1
  Abs/1 -> 1-D Lookup Table/1
  1-D Lookup Table1/1 -> Product/1
  gain1/1 -> Product1/1

== system METI_Thermal_ver01_Jmaab_2018b/Vehicle/TM_PNT/TM_PNT/TC_PNT/LU_Clutch ==
  note: クラッチモデル
      | LockUp ON時は硬いバネダンパー、OFF時はトルク0 Nm
  LockUP_Signal : Inport
  w_TM_PNT_in_radps1 : Inport  Port=2
  w_TM_PNT_in_radps2 : Inport  Port=3
  Gain1 : Gain  Gain=TM_PNT_Gain_LU_spring_Nmprad
  Gain2 : Gain  Gain=TM_PNT_Gain_LU_damper_Nmsprad
  Integrator : Integrator  ExternalReset=level  LimitOutput=on  UpperSaturationLimit=1  LowerSaturationLimit=-1
  Logical Operator : Logic  Operator=NOT  AllPortsSameDT=off  OutDataTypeStr=boolean
  Product : Product  RndMeth=Zero
  Product2 : Product  RndMeth=Zero
  Sum1 : Sum  Inputs=|+-
  Sum2 : Sum  Inputs=++|
  Transfer Fcn : TransferFcn  Denominator=[TM_PNT_tau_LU_Clutch_s 1]
  trq_LUC_Nm1 : Outport
  trq_LUC_Nm2 : Outport  Port=2
  wires:
  w_TM_PNT_in_radps1/1 -> Product/2
  LockUP_Signal/1 -> Logical Operator/1, Transfer Fcn/1
  Sum2/1 -> trq_LUC_Nm2/1, trq_LUC_Nm1/1
  Product2/1 -> Sum1/2
  Product/1 -> Sum1/1
  Integrator/1 -> Gain1/1
  Sum1/1 -> Integrator/1, Gain2/1
  Transfer Fcn/1 -> Product2/1, Product/1
  w_TM_PNT_in_radps2/1 -> Product2/2
  Logical Operator/1 -> Integrator/2
  Gain1/1 -> Sum2/2
  Gain2/1 -> Sum2/1

== system METI_Thermal_ver01_Jmaab_2018b/Vehicle/TM_PNT/TM_PNT/TC_PNT/T_C ==
  w_TM_PNT_in_radps1 : Inport
  w_TM_PNT_in_radps2 : Inport  Port=2
  Cal_C_Capacity : Subsystem
  Cal_Ratio_n : Subsystem
  Cal_trq_TC_eng : Subsystem
  Gain : Gain  Gain=radpsec2rpm
  Gain1 : Gain  Gain=radpsec2rpm
  Product1 : Product  RndMeth=Zero
  トルク比 Lookup Table2 : Lookup_n-D  NumberOfTableDimensions=1  BreakpointsForDimension1=TM_PNT_torque_ratio_table_x_speed_ratio  Table=TM_PNT_torque_ratio_table  ExtrapMethod=Clip  RndMeth=Simplest  InputSameDT=on
  trq_TC_Nm1 : Outport
  trq_TC_Nm2 : Outport  Port=2
  wires:
  Gain/1 -> Cal_Ratio_n/2(n_GR_rpm)  "n_GR_rpm"
  Gain1/1 -> Cal_Ratio_n/1(n_TM_PNT_rpm), Cal_trq_TC_eng/1("n_TM_PNT_rpm ")  "n_TM_PNT_rpm"
  w_TM_PNT_in_radps2/1 -> Gain/1
  Product1/1 -> trq_TC_Nm1/1
  トルク比 Lookup Table2/1 -> Product1/2
  w_TM_PNT_in_radps1/1 -> Gain1/1
  Cal_Ratio_n/1(ratio_n) -> トルク比 Lookup Table2/1, Cal_C_Capacity/1(ratio_n)
  Cal_trq_TC_eng/1(trq_TC_Nm) -> trq_TC_Nm2/1, Product1/1  "trq_TC_Nm"
  Cal_C_Capacity/1(c_capacity) -> Cal_trq_TC_eng/2(c_capacity)
  Cal_Ratio_n/2(flag_acc_del) -> Cal_C_Capacity/2(flag_acc_del)

== system METI_Thermal_ver01_Jmaab_2018b/Vehicle/CNT/ENG_CNT/ENG_Cntrl/Caliculate_Idle_Speed/Subsystem ==
  del_omg_engine : Inport
  flag_idle_fb : Inport  Port=2
  Gain : Gain  Gain=ENG_CNT_gain_p_per_isc
  Logical Operator1 : Logic  Operator=NOT  AllPortsSameDT=off  OutDataTypeStr=boolean
  Memory : Memory  InitialCondition=4
  Saturation : Saturate  UpperLimit=ENG_CNT_per_isc_max  LowerLimit=ENG_CNT_per_isc_min
  Switch : Switch  Criteria=u2 > Threshold  Threshold=0.5
  per_isc_[%] : Outport
  wires:
  Switch/1 -> Saturation/1
  flag_idle_fb/1 -> Logical Operator1/1
  Gain/1 -> Switch/3
  Memory/1 -> Switch/1
  Saturation/1 -> per_isc_[%]/1, Memory/1
  del_omg_engine/1 -> Gain/1
  Logical Operator1/1 -> Switch/2
